simulink model "emp"  (R2020b)
settings: Solver=VariableStepAuto  StartTime=0.0  StopTime=10.0  RelTol=1e-3
settings Model: Creator=morro  LastModifiedBy=morro

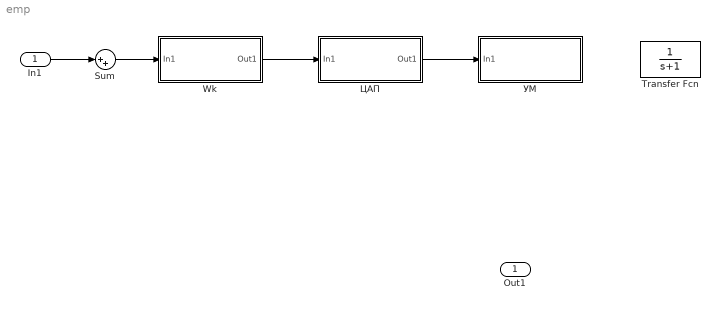
== system emp ==
  In1 : Inport
  Sum : Sum  Inputs=|++
  Transfer Fcn : TransferFcn  Denominator=[1 1]
  Wk : Subsystem  TreatAsAtomicUnit=on
  УМ : Subsystem  TreatAsAtomicUnit=on
  ЦАП : Subsystem  TreatAsAtomicUnit=on
  Out1 : Outport
  wires:
  Sum/1 -> Wk/1(In1)
  Wk/1(Out1) -> ЦАП/1(In1)
  ЦАП/1(Out1) -> УМ/1(In1)
  In1/1 -> Sum/1

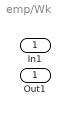
== system emp/Wk ==
  In1 : Inport
  Out1 : Outport

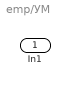
== system emp/УМ ==
  In1 : Inport

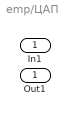
== system emp/ЦАП ==
  In1 : Inport
  Out1 : Outport
